simulink model "WhippleModel_dis"  (R2018a)
settings: Solver=VariableStepAuto  StartTime=0.0  StopTime=7  MaxStep=0.01  RelTol=1e-3
values from neighbouring files (symbols this model uses):
  sys_Whipple_dis = c2d(sys_Whipple_cont,Ts)    [DynamicModelParameters.m]
libraries: simulink_extras x2, simulink x1
settings Model: Creator=ProjectHT2018-2  LastModifiedBy=Tom
settings DebuggingCC: LibraryContextMissingDiagnostic=warning
settings SFSimCC: SimUseLocalCustomCode=on
settings RTWCC: RTWUseLocalCustomCode=on

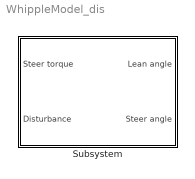
== system WhippleModel_dis ==
  Subsystem : Subsystem

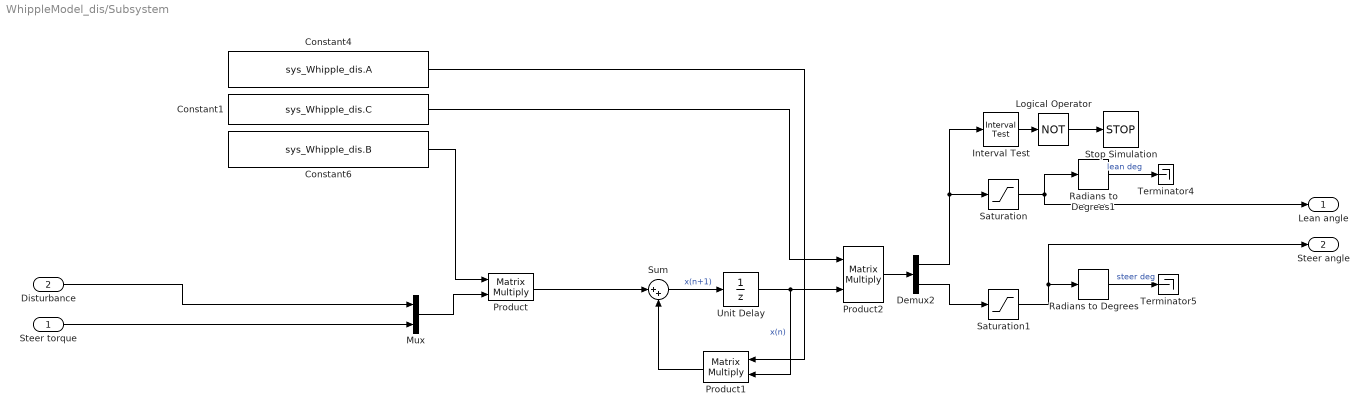
== system WhippleModel_dis/Subsystem ==
  Steer torque : Inport
  Disturbance : Inport  Port=2
  Constant1 : Constant  Value=sys_Whipple_dis.C
  Constant4 : Constant  Value=sys_Whipple_dis.A
  Constant6 : Constant  Value=sys_Whipple_dis.B
  Demux2 : Demux  Outputs=2
  Interval Test : simulink/Logic and Bit Operations/Interval Test  IntervalClosedRight=on  uplimit=pi/4  IntervalClosedLeft=on  lowlimit=-pi/4  OutDataTypeStr=boolean
  Logical Operator : Logic  Operator=NOT  AllPortsSameDT=off  OutDataTypeStr=boolean
  Mux : Mux  Inputs=2
  Product : Product  Multiplication=Matrix(*)
  Product1 : Product  Multiplication=Matrix(*)
  Product2 : Product  Multiplication=Matrix(*)
  Radians to Degrees : simulink_extras/Transformations/Radians to Degrees
  Radians to Degrees1 : simulink_extras/Transformations/Radians to Degrees
  Saturation : Saturate  UpperLimit=pi/2  LowerLimit=-pi/2
  Saturation1 : Saturate  UpperLimit=pi/2  LowerLimit=-pi/2
  Stop Simulation : Stop
  Sum : Sum  Inputs=|++
  Terminator4 : Terminator
  Terminator5 : Terminator
  Unit Delay : UnitDelay  SampleTime=-1
  "Lean angle " : Outport
  Steer angle : Outport  Port=2
  wires:
  Constant1/1 -> Product2/1
  Mux/1 -> Product/2
  Disturbance/1 -> Mux/1
  Product/1 -> Sum/1
  Steer torque/1 -> Mux/2
  Demux2/2 -> Saturation1/1
  Constant6/1 -> Product/1
  Saturation1/1 -> Steer angle/1, Radians to Degrees/1
  Interval Test/1 -> Logical Operator/1
  Sum/1 -> Unit Delay/1  "x(n+1)"
  Radians to Degrees/1 -> Terminator5/1  "steer deg"
  Saturation/1 -> "Lean angle "/1, Radians to Degrees1/1
  Demux2/1 -> Interval Test/1, Saturation/1
  Product2/1 -> Demux2/1
  Unit Delay/1 -> Product1/2, Product2/2  "x(n)"
  Product1/1 -> Sum/2
  Constant4/1 -> Product1/1
  Logical Operator/1 -> Stop Simulation/1
  Radians to Degrees1/1 -> Terminator4/1  "lean deg"
